simulink model "Copy_of_PredictiveSim"  (R2020b)
settings: Solver=VariableStepAuto  StartTime=0.0  StopTime=801  RelTol=1e-3
undefined symbols (not defined in the file or in its folder): threshold
libraries: simulink x1, deeplib x1
settings Model: Creator=Alia  LastModifiedBy=Alia

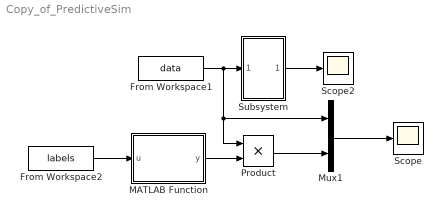
== system Copy_of_PredictiveSim ==
  From Workspace1 : FromWorkspace  VariableName=data
  From Workspace2 : FromWorkspace  VariableName=labels
  MATLAB Function : MATLAB Function  TreatAsAtomicUnit=on
  Mux1 : Mux  Inputs=2
  Product : Product
  Scope : Scope
  Scope2 : Scope
  Subsystem : Subsystem  mask{BufferLength=50, NetworkFilePath=C:\Users\Alia\Desktop\idriss\net.mat}
      mask prompts: BufferLength "dspshared:blkprm_prompts:OutputBufferSize"; NetworkFilePath "deep_blocks:common:FilePath"
      mask help: Buffer overload value must be equal to 1-BufferSize
      mask TypeOptions BufferLength:
      | Buffer/N | Delay/DelayLength | Compare
      | To Constant/const
      mask TypeOptions NetworkFilePath: Predict1/NetworkFilePath
      mask DialogControl BufferLength Prompt: Output buffer size (per channel):
      mask DialogControl NetworkFilePath Prompt: File path:
  wires:
  From Workspace2/1 -> MATLAB Function/1(u)
  Product/1 -> Mux1/2
  MATLAB Function/1(y) -> Product/2
  Subsystem/1(Out1) -> Scope2/1
  From Workspace1/1 -> Mux1/1, Product/1, Subsystem/1(In1)
  Mux1/1 -> Scope/1

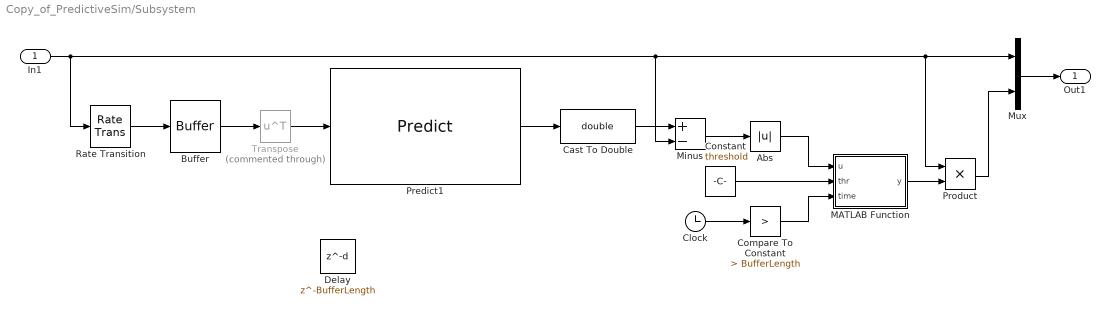
== system Copy_of_PredictiveSim/Subsystem ==
  In1 : Inport
  Abs : Abs
  Buffer : Buffer  N=BufferLength  V=BufferLength-1  OutputFrames=off
  Cast To Double : DataTypeConversion  OutDataTypeStr=double
  Clock : Clock
  Compare To Constant : simulink/Logic and Bit Operations/Compare To Constant  relop=>  const=BufferLength  OutDataTypeStr=boolean
  Constant : Constant  Value=threshold
  Delay : Delay  DelayLength=BufferLength  SampleTime=1
  MATLAB Function : MATLAB Function  TreatAsAtomicUnit=on
  Minus : Sum  Inputs=+-
  Mux : Mux  Inputs=2
  Predict1 : deeplib/Predict  Network=Network from MAT-file  NetworkFunction=squeezenet  NetworkFilePath=C:\Users\Alia\Desktop\idriss\net.mat  MiniBatchSize=128  InputDataFormats={ '', '' }  Predictions=on  Activations={}  ForceInterpretedSim=off  EnableDLNetwork=off
      settings: SourceProductBaseCode=NN
  Product : Product
  Rate Transition : RateTransition  OutPortSampleTime=1
  Transpose : Math  Commented=through  Operator=transpose  SaturateOnIntegerOverflow=on
  Out1 : Outport
  wires:
  Clock/1 -> Compare To Constant/1
  Product/1 -> Mux/2
  Buffer/1 -> Transpose/1
  MATLAB Function/1(y) -> Product/2
  Compare To Constant/1 -> MATLAB Function/3(time)
  Cast To Double/1 -> Minus/1
  Transpose/1 -> Predict1/1
  Constant/1 -> MATLAB Function/2(thr)
  Rate Transition/1 -> Buffer/1
  Minus/1 -> Abs/1
  Abs/1 -> MATLAB Function/1(u)
  Predict1/1 -> Cast To Double/1
  Mux/1 -> Out1/1
  In1/1 -> Product/1, Mux/1, Minus/2, Rate Transition/1

== matlab function Copy_of_PredictiveSim/MATLAB Function ==
  data: u input; y output
function y = fcn(u)
y = NaN;
if u == 1
    y = 1;
end

== matlab function Copy_of_PredictiveSim/Subsystem/MATLAB Function ==
  data: u input; y output; thr input; time input
function y = fcn(u,thr, time)
y = NaN;
if time == 1
    if u > thr
    y = 1;
    end
end
